simulink model "CAVE_MachE_sil_test_v2"  (R2019b)
settings: configuration reference "ConfigSetDesktopFixedStep" (kept outside this file)
PreLoadFcn:
  | VSS_BICYCLE=Simulink.Variant('Dual=0');
  | VSS_DUAL=Simulink.Variant('Dual=1');
  | Dual=1;
  | load('DriveCycle2.mat')
PostLoadFcn:
  | if any(exist('dsrtsu_mdlpostloadfcn', 'file') ~= 0), dsrtsu_mdlpostloadfcn('Execute', bdroot); end
InitFcn:
  | , if any(exist('dsmpb_private', 'file') ~= 0), dsmpb_private('dsmpb_mdlclblib', 'Init', bdroot); end,
  | load('DriveCycle2.mat')
model workspace (MAT data in the model file):
  Gas = 0.383333333333
values from neighbouring files (symbols this model uses):
  CoastDown =     [Run_Simulink.mat]
  limitedMCT =     [Run_Simulink.mat]
  MCT =     [Run_Simulink.mat]
  pMCT =     [Run_Simulink.mat]
  US06 =     [Run_Simulink.mat]
undefined symbols (not defined in the file or in its folder): AccelCmd, ActTqLF_Nm_, ActTqLR_Nm_, ActTqRF_Nm_, ActTqRR_Nm_, BattChargeLimitMaxPwr, BattChargeLimitSocBpts, BattChargeLimitTbl, BattChrgCapcty, BattDischargeLimitSocBpts, BattDischargeLimitTbl, BattDischargeMaxPwr, BattNumCellsParallel, BattNumCellsSeries, BattOpenVoltCapBpts, BattOpenVoltTbl, BattResistSocBpts, BattResistTbl, BattResistTempBpts, BrakeMaxPrs, BrakeMaxTrq, ChassisDistCg2FrontAxle, ChassisDistCg2RearAxle, ChassisVehMass, CltchCmd, DecelCmd, DiffRatio, DiscIntNeverNeededParam, EnvGravCnst, EnvPrs, EnvTemp, FuelSpecificGrav, GearCmd, h, InitStates, lgSw, MtrEffSpdBpts, MtrEffTbl, MtrEffTrqBpts, MtrPwrMax, MtrTrqMax, SteeringCmd, SupvsryCtrlRegenBrkCutOffTbl, SupvsryCtrlRegenSpdBpts, TestScnrioCycleNum, VEH
libraries: VSIGenLib x39, simulink x27, etargetslib x24, CarMaker4SL x8, vehdynlibtire x8, vehdynlibsuspension x7, vehdynlibtirecommon x7, autolibutils x5, autolibshared x5, VsrLibWheel x4, autolibpowerinfoutils x3, sharedtransform x3
(part 1 of 12)
PreSaveFcn:
  | , if any(exist('dsmpb_private', 'file') ~= 0), dsmpb_private('dsmpb_mdlclblib', 'PreSave', bdroot); end,
CloseFcn:
  | , if any(exist('dsmpb_private', 'file') ~= 0), dsmpb_private('dsmpb_mdlclblib', 'Close', bdroot); end,
settings Model: DataDictionary=DdPassengerEv.sldd  EnableAccessToBaseWorkspace=off  DSMPB_ID_DATA={'19138',struct('BlockId','c43ab22d-bd8f-46e8-9c1b-50244a2b4c3c','SignalIds',{{'677ec428-0e4b-4948-912c-2a0f547451ce'}}),'19214',struct('BlockId','c6d59404-7243-491d-a0f6-53a7c58573d2','SignalIds',{{'1bb5ce4d-6ca7-438d-a7c7-83dc6b8f8ba2','d23deae5-7b45-4d37-a8c2-65a1bc4ec57e','d73ea5da-e326-4b10-9ae8-bf6dd5d0d571','a3187cc6-40b5-42b9-9fee-06cfa4cf2657','616fd28a-17a3-40f5-a1a4-f6fdafbaa436'}})}  RTICANMMDATA=struct('GeneralSetupData',struct('modelroot','C:\GitDev\Anye\cave_carla_dev\Vehicles\VehicleProjects\Bolt_EV\System','generalsettings',struct('filesettings',struct('destfolder',struct('Name','RTICANMM_FILES','Check',1),'buildfolder',struct('Name','.','Check',1),'AbsDestfolder',struct('Name','C:\GitDev\Anye\cave_carla_dev\Vehicles\VehicleProjects\Bolt_EV\System\RTICANMM_FILES'),'AbsBuildfolder',struct('Name','C:\GitDev\Anye\cave_carla_dev\Vehicles\VehicleProjects\Bolt_EV\System'))),'options',struct('addpaths',1,'rmpaths',1,'addtrcexclusion',true,'cannavigator',struct('checkmonitoring',0),'show_usrtrc',0,'use_usrtrc',0),'advanced',struct('options',ones(1,100)),'MPSetup',{{}},'RTI',struct('Type','DSRT','Ver','4.2p1','Date','11-Feb-2020'),'modelname','CAVE_MachE_sil_test_v2','block','CAVE_MachE_sil_test_v2'))  DSRTSU_INTERNAL_RTIFPGA=150  PauseTimes=45  OrderedModelArguments=off  Creator=9bt  LastModifiedBy=RVDP
settings ConfigSetRef: SourceName=ConfigSetDesktopFixedStep

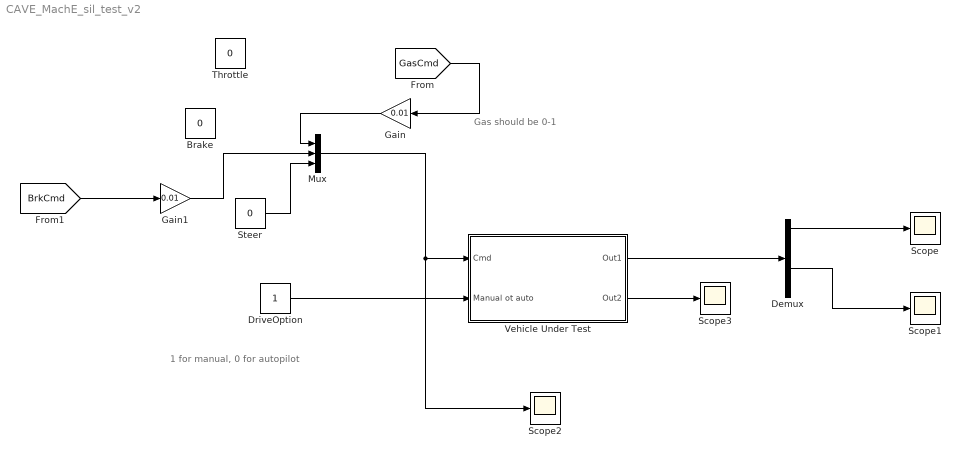
== system CAVE_MachE_sil_test_v2 ==
  note: 1 for manual, 0 for autopilot
  note: Gas should be 0-1
  Brake : Constant  Value=0
  Demux : Demux
  DriveOption : Constant
  Gain : Gain  Gain=0.01
  Gain1 : Gain  Gain=0.01
  Mux : Mux  Inputs=3
  Scope{,1..3} (4 alike) : Scope
  Steer : Constant  Value=0
  Throttle : Constant  Value=0
  Vehicle Under Test : Subsystem
  wires:
  Vehicle Under Test/1(Out1) -> Demux/1
  Demux/1 -> Scope/1
  Mux/1 -> Scope2/1, Vehicle Under Test/1(Cmd)
  Demux/3 -> Scope1/1
  Vehicle Under Test/2(Out2) -> Scope3/1
  DriveOption/1 -> Vehicle Under Test/2(Manual ot auto)
  [GasCmd] -> Gain/1
  [BrkCmd] -> Gain1/1
  Steer/1 -> Mux/3
  Gain1/1 -> Mux/2
  Gain/1 -> Mux/1

== system CAVE_MachE_sil_test_v2/Vehicle Under Test ==
  Cmd : Inport
  Manual ot auto : Inport  Port=2
  AccelCmdOutput_Anye : Terminator
  Ackerman steer : Lookup_n-D  NumberOfTableDimensions=1  BreakpointsForDimension1="[-0.446316297916244\t-0.442150786830951\t-0.437977161945005\t-0.433795286969319\t-0.429605025209166\t-0.425406239561593\t-0.421198792513030\t-0.416982546137136\t-0.412757362092861\t-0.408523101622746\t-0.404279625551461\t-0.400026794284603\t-0.395764467807732\t-0.391492505685692\t-0.387210767062193\t-0.382919110659678\t-0.378617394779480\t-0.374305477302279\t-0.369983215688866\t-0.365650466981227\t-0.361307087803951\t-0.356952934365975\t-0.352587862462675\t-0.348211727478321\t-0.343824384388886\t-0.339425687765245\t-0.335015491776758\t-0.330593650195247\t-0.326160016399396\t-0.321714443379563\t-0.317256783743034\t-0.312786889719717\t-0.308304613168298\t-0.303809805582871\t-0.299302318100048\t-0.294782001506567\t-0.290248706247410\t-0.285702282434450\t-0.281142579855627\t-0.276569447984685\t-0.271982735991464\t-0.267382292752788\t-0.262767966863931\t-0.258139606650706\t-0.253497060182174\t-0.248840175283994\t-0.244168799552432\t-0.239482780369037\t-0.234781964916014\t-0.230066200192295\t-0.225335333030331\t-0.220589210113630\t-0.215827677995039\t-0.211050583115807\t-0.206257771825433\t-0.201449090402323\t-0.196624385075265\t-0.191783502045761\t-0.186926287511198\t-0.182052587688919\t-0.177162248841170\t-0.172255117300976\t-0.167331039498945\t-0.162389861991014\t-0.157431431487183\t-0.152455594881217\t-0.147462199281363\t-0.142451092042095\t-0.137422120796894\t-0.132375133492088\t-0.127309978421782\t-0.122226504263869\t-0.117124560117169\t-0.112003995539695\t-0.106864660588066\t-0.101706405858090\t-0.0965290825265349\t-0.0913325423940914\t-0.0861166379295599\t-0.0808812223152671\t-0.0756261494937309\t-0.0703512742155897\t-0.0650564520888085\t-0.0597415396291770\t-0.0544063943121130\t-0.0490508746257825\t-0.0436748401255510\t-0.0382781514897739\t-0.0328606705769398\t-0.0274222604841732\t-0.0219627856071077\t-0.0164821117011354\t-0.0109801059440403\t-0.00545663700002112\t0\t0.00547767577609933\t0.0110656090794470\t0.0166755107772618\t0.0223075038233658\t0.0279617092740365\t0.0336382462142580\t0.0393372316825870\t0.0450587805946413\t0.0508030056652199\t0.0565700173290652\t0.0623599236602815\t0.0681728302904245\t0.0740088403252790\t0.0798680542603446\t0.0857505698950509\t0.0916564822457268\t0.0975858834573503\t0.103538862714108\t0.109515506148794\t0.115515896751090\t0.121540114274751\t0.127588235143750\t0.133660332357415\t0.139756475394610\t0.145876730117007\t0.152021158671496\t0.158189819391799\t0.164382766699339\t0.170600051003425\t0.176841718600822\t0.183107811574771\t0.189398367693541\t0.195713420308563\t0.202052998252265\t0.208417125735647\t0.214805822245717\t0.221219102442855\t0.227656976058216\t0.234119447791246\t0.240606517207442\t0.247118178636427\t0.253654421070478\t0.260215228063589\t0.266800577631217\t0.273410442150791\t0.280044788263140\t0.286703576774936\t0.293386762562311\t0.300094294475738\t0.306826115246357\t0.313582161393837\t0.320362363135953\t0.327166644299990\t0.333994922236136\t0.340847107733006\t0.347723104935443\t0.354622811264752\t0.361546117341510\t0.368492906911125\t0.375463056772267\t0.382456436708368\t0.389472909422305\t0.396512330474460\t0.403574548224288\t0.410659403775562\t0.417766730925451\t0.424896356117582\t0.432048098399246\t0.439221769382891\t0.446417173212069\t0.453634106531970\t0.460872358464695\t0.468131710589418\t0.475411936927561\t0.482712803933137\t0.490034070488372\t0.497375487904758\t0.504736799929627\t0.512117742758400\t0.519518045052588\t0.526937427963674\t0.534375605162959\t0.541832282877473\t0.549307159932028\t0.556799927797496\t0.564310270645373\t0.571837865408689\t0.579382381849329\t0.586943482631776\t0.594520823403350\t0.602114052880920\t0.609722812944144\t0.617346738735206\t0.624985458765058]"  Table="[-9.40000000000000\t-9.30000000000000\t-9.20000000000000\t-9.10000000000000\t-9\t-8.90000000000000\t-8.80000000000000\t-8.70000000000000\t-8.60000000000000\t-8.50000000000000\t-8.40000000000000\t-8.30000000000000\t-8.20000000000000\t-8.10000000000000\t-8\t-7.90000000000000\t-7.80000000000000\t-7.70000000000000\t-7.60000000000000\t-7.50000000000000\t-7.40000000000000\t-7.30000000000000\t-7.20000000000000\t-7.10000000000000\t-7\t-6.90000000000000\t-6.80000000000000\t-6.70000000000000\t-6.60000000000000\t-6.50000000000000\t-6.40000000000000\t-6.30000000000000\t-6.20000000000000\t-6.10000000000000\t-6\t-5.90000000000000\t-5.80000000000000\t-5.70000000000000\t-5.60000000000000\t-5.50000000000000\t-5.40000000000000\t-5.30000000000000\t-5.20000000000000\t-5.10000000000000\t-5\t-4.90000000000000\t-4.80000000000000\t-4.70000000000000\t-4.60000000000000\t-4.50000000000000\t-4.40000000000000\t-4.30000000000000\t-4.20000000000000\t-4.10000000000000\t-4\t-3.90000000000000\t-3.80000000000000\t-3.70000000000000\t-3.60000000000000\t-3.50000000000000\t-3.40000000000000\t-3.30000000000000\t-3.20000000000000\t-3.10000000000000\t-3\t-2.90000000000000\t-2.80000000000000\t-2.70000000000000\t-2.60000000000000\t-2.50000000000000\t-2.40000000000000\t-2.30000000000000\t-2.20000000000000\t-2.10000000000000\t-2\t-1.90000000000000\t-1.80000000000000\t-1.70000000000000\t-1.60000000000000\t-1.50000000000000\t-1.40000000000000\t-1.30000000000000\t-1.20000000000000\t-1.10000000000000\t-1\t-0.900000000000000\t-0.800000000000000\t-0.700000000000000\t-0.600000000000000\t-0.500000000000000\t-0.400000000000000\t-0.300000000000000\t-0.200000000000000\t-0.100000000000000\t0\t0.100000000000000\t0.200000000000000\t0.300000000000000\t0.400000000000000\t0.500000000000000\t0.600000000000000\t0.700000000000000\t0.800000000000000\t0.900000000000000\t1\t1.10000000000000\t1.20000000000000\t1.30000000000000\t1.40000000000000\t1.50000000000000\t1.60000000000000\t1.70000000000000\t1.80000000000000\t1.90000000000000\t2\t2.10000000000000\t2.20000000000000\t2.30000000000000\t2.40000000000000\t2.50000000000000\t2.60000000000000\t2.70000000000000\t2.80000000000000\t2.90000000000000\t3\t3.10000000000000\t3.20000000000000\t3.30000000000000\t3.40000000000000\t3.50000000000000\t3.60000000000000\t3.70000000000000\t3.80000000000000\t3.90000000000000\t4\t4.10000000000000\t4.20000000000000\t4.30000000000000\t4.40000000000000\t4.50000000000000\t4.60000000000000\t4.70000000000000\t4.80000000000000\t4.90000000000000\t5\t5.10000000000000\t5.20000000000000\t5.30000000000000\t5.40000000000000\t5.50000000000000\t5.60000000000000\t5.70000000000000\t5.80000000000000\t5.90000000000000\t6\t6.10000000000000\t6.20000000000000\t6.30000000000000\t6.40000000000000\t6.50000000000000\t6.60000000000000\t6.70000000000000\t6.80000000000000\t6.90000000000000\t7\t7.10000000000000\t7.20000000000000\t7.30000000000000\t7.40000000000000\t7.50000000000000\t7.60000000000000\t7.70000000000000\t7.80000000000000\t7.90000000000000\t8\t8.10000000000000\t8.20000000000000\t8.30000000000000\t8.40000000000000\t8.50000000000000\t8.60000000000000\t8.70000000000000\t8.80000000000000\t8.90000000000000\t9\t9.10000000000000\t9.20000000000000\t9.30000000000000\t9.40000000000000]"  InternalRulePriority=Speed  RndMeth=Simplest  InputSameDT=on
  Bus Creator : BusCreator  Inputs=AccelCmd,DecelCmd,GearCmd,CltchCmd,lgSw,SteeringCmd
  Bus Creator1 : BusCreator  Inputs=8
  Bus Creator2 : BusCreator  Inputs=2
  Bus Selector : BusSelector  OutputSignals=Veh.Chassis.X,Veh.Chassis.Y,Veh.Chassis.psi,Veh.Batt.BattSoc,Veh.Batt.BattCurr,Veh.Batt.BattVolt,Veh.Diff.Axl1.Axl1Trq,Veh.Chassis.VehSpd
  Clock : Clock
  Constant : Constant  Value=0
  Constant1 : Constant  Value=0  SampleTime=0.001
  Constant2 : Constant
  Constant3 : Constant  Value=0
  Constant4 : Constant
  Constant6 : Constant  Value=0.5  SampleTime=0.001
  Demux : Demux  Outputs=3
  EV Bolt Steer : Lookup_n-D  NumberOfTableDimensions=1  BreakpointsForDimension1="[-0.541571931581492\t-0.535619550629112\t-0.529667169676731\t-0.523714788724350\t-0.517762407771969\t-0.511810026819588\t-0.505857645867207\t-0.499905264914826\t-0.493952883962445\t-0.488000503010064\t-0.482048122057683\t-0.476095741105302\t-0.470143360152921\t-0.464190979200541\t-0.458238598248160\t-0.452286217295779\t-0.446333836343398\t-0.440381455391017\t-0.434429074438636\t-0.428476693486255\t-0.422524312533874\t-0.416571931581493\t-0.410619550629112\t-0.404667169676731\t-0.398714788724350\t-0.392762407771969\t-0.386810026819588\t-0.380857645867207\t-0.374905264914826\t-0.368952883962445\t-0.363000503010064\t-0.357048122057683\t-0.351095741105302\t-0.345143360152921\t-0.339190979200541\t-0.333238598248160\t-0.327286217295779\t-0.321333836343398\t-0.315381455391017\t-0.309429074438636\t-0.303476693486255\t-0.297524312533874\t-0.291571931581493\t-0.285619550629112\t-0.279667169676731\t-0.273714788724350\t-0.267762407771969\t-0.261810026819588\t-0.255857645867207\t-0.249905264914826\t-0.243952883962445\t-0.238000503010065\t-0.232048122057684\t-0.226095741105303\t-0.220143360152922\t-0.214190979200541\t-0.208238598248160\t-0.202286217295779\t-0.196333836343398\t-0.190381455391017\t-0.184429074438636\t-0.178476693486255\t-0.172524312533874\t-0.166571931581493\t-0.160619550629112\t-0.154667169676731\t-0.148714788724350\t-0.142762407771969\t-0.136810026819588\t-0.130857645867207\t-0.124905264914826\t-0.118952883962445\t-0.113000503010064\t-0.107048122057683\t-0.101095741105303\t-0.0951433601529216\t-0.0891909792005406\t-0.0832385982481596\t-0.0772862172957787\t-0.0713338363433977\t-0.0653814553910168\t-0.0594290744386358\t-0.0534766934862548\t-0.0475243125338739\t-0.0415719315814929\t-0.0356195506291120\t-0.0296671696767310\t-0.0237147887243500\t-0.0177624077719691\t-0.0118100268195881\t-0.00585764586720720\t0\t0.00585764586720720\t0.0118100268195881\t0.0177624077719691\t0.0237147887243500\t0.0296671696767310\t0.0356195506291120\t0.0415719315814929\t0.0475243125338739\t0.0534766934862548\t0.0594290744386358\t0.0653814553910168\t0.0713338363433977\t0.0772862172957787\t0.0832385982481596\t0.0891909792005406\t0.0951433601529216\t0.101095741105303\t0.107048122057683\t0.113000503010064\t0.118952883962445\t0.124905264914826\t0.130857645867207\t0.136810026819588\t0.142762407771969\t0.148714788724350\t0.154667169676731\t0.160619550629112\t0.166571931581493\t0.172524312533874\t0.178476693486255\t0.184429074438636\t0.190381455391017\t0.196333836343398\t0.202286217295779\t0.208238598248160\t0.214190979200541\t0.220143360152922\t0.226095741105303\t0.232048122057684\t0.238000503010065\t0.243952883962445\t0.249905264914826\t0.255857645867207\t0.261810026819588\t0.267762407771969\t0.273714788724350\t0.279667169676731\t0.285619550629112\t0.291571931581493\t0.297524312533874\t0.303476693486255\t0.309429074438636\t0.315381455391017\t0.321333836343398\t0.327286217295779\t0.333238598248160\t0.339190979200541\t0.345143360152921\t0.351095741105302\t0.357048122057683\t0.363000503010064\t0.368952883962445\t0.374905264914826\t0.380857645867207\t0.386810026819588\t0.392762407771969\t0.398714788724350\t0.404667169676731\t0.410619550629112\t0.416571931581493\t0.422524312533874\t0.428476693486255\t0.434429074438636\t0.440381455391017\t0.446333836343398\t0.452286217295779\t0.458238598248160\t0.464190979200541\t0.470143360152921\t0.476095741105302\t0.482048122057683\t0.488000503010064\t0.493952883962445\t0.499905264914826\t0.505857645867207\t0.511810026819588\t0.517762407771969\t0.523714788724350\t0.529667169676731\t0.535619550629112\t0.541571931581492]"  Table="[-9.10000000000000\t-9\t-8.90000000000000\t-8.80000000000000\t-8.70000000000000\t-8.60000000000000\t-8.50000000000000\t-8.40000000000000\t-8.30000000000000\t-8.20000000000000\t-8.10000000000000\t-8\t-7.90000000000000\t-7.80000000000000\t-7.70000000000000\t-7.60000000000000\t-7.50000000000000\t-7.40000000000000\t-7.30000000000000\t-7.20000000000000\t-7.10000000000000\t-7\t-6.90000000000000\t-6.80000000000000\t-6.70000000000000\t-6.60000000000000\t-6.50000000000000\t-6.40000000000000\t-6.30000000000000\t-6.20000000000000\t-6.10000000000000\t-6\t-5.90000000000000\t-5.80000000000000\t-5.70000000000000\t-5.60000000000000\t-5.50000000000000\t-5.40000000000000\t-5.30000000000000\t-5.20000000000000\t-5.10000000000000\t-5\t-4.90000000000000\t-4.80000000000000\t-4.70000000000000\t-4.60000000000000\t-4.50000000000000\t-4.40000000000000\t-4.30000000000000\t-4.20000000000000\t-4.10000000000000\t-4\t-3.90000000000000\t-3.80000000000000\t-3.70000000000000\t-3.60000000000000\t-3.50000000000000\t-3.40000000000000\t-3.30000000000000\t-3.20000000000000\t-3.10000000000000\t-3\t-2.90000000000000\t-2.80000000000000\t-2.70000000000000\t-2.60000000000000\t-2.50000000000000\t-2.40000000000000\t-2.30000000000000\t-2.20000000000000\t-2.10000000000000\t-2\t-1.90000000000000\t-1.80000000000000\t-1.70000000000000\t-1.60000000000000\t-1.50000000000000\t-1.40000000000000\t-1.30000000000000\t-1.20000000000000\t-1.10000000000000\t-1\t-0.900000000000000\t-0.800000000000000\t-0.700000000000000\t-0.600000000000000\t-0.500000000000000\t-0.400000000000000\t-0.300000000000000\t-0.200000000000000\t-0.100000000000000\t0\t0.100000000000000\t0.200000000000000\t0.300000000000000\t0.400000000000000\t0.500000000000000\t0.600000000000000\t0.700000000000000\t0.800000000000000\t0.900000000000000\t1\t1.10000000000000\t1.20000000000000\t1.30000000000000\t1.40000000000000\t1.50000000000000\t1.60000000000000\t1.70000000000000\t1.80000000000000\t1.90000000000000\t2\t2.10000000000000\t2.20000000000000\t2.30000000000000\t2.40000000000000\t2.50000000000000\t2.60000000000000\t2.70000000000000\t2.80000000000000\t2.90000000000000\t3\t3.10000000000000\t3.20000000000000\t3.30000000000000\t3.40000000000000\t3.50000000000000\t3.60000000000000\t3.70000000000000\t3.80000000000000\t3.90000000000000\t4\t4.10000000000000\t4.20000000000000\t4.30000000000000\t4.40000000000000\t4.50000000000000\t4.60000000000000\t4.70000000000000\t4.80000000000000\t4.90000000000000\t5\t5.10000000000000\t5.20000000000000\t5.30000000000000\t5.40000000000000\t5.50000000000000\t5.60000000000000\t5.70000000000000\t5.80000000000000\t5.90000000000000\t6\t6.10000000000000\t6.20000000000000\t6.30000000000000\t6.40000000000000\t6.50000000000000\t6.60000000000000\t6.70000000000000\t6.80000000000000\t6.90000000000000\t7\t7.10000000000000\t7.20000000000000\t7.30000000000000\t7.40000000000000\t7.50000000000000\t7.60000000000000\t7.70000000000000\t7.80000000000000\t7.90000000000000\t8\t8.10000000000000\t8.20000000000000\t8.30000000000000\t8.40000000000000\t8.50000000000000\t8.60000000000000\t8.70000000000000\t8.80000000000000\t8.90000000000000\t9\t9.10000000000000]"  InternalRulePriority=Speed  RndMeth=Simplest  InputSameDT=on
  Environment : Subsystem
  Monitor : Subsystem
  Step : Step  Time=3  After=0
  Switch : Switch  Criteria=u2 > Threshold
  Switch1 : Switch  Criteria=u2 > Threshold
  Switch2 : Switch  Criteria=u2 > Threshold
  To Workspace : ToWorkspace  VariableName=EvBoltCalib  SaveFormat=Structure With Time  SampleTime=-1
  Vector Concatenate : Concatenate  NumInputs=4
  Vehicle : Subsystem
  Out1 : Outport
  Out2 : Outport  Port=2
  wires:
  Bus Creator2/1 -> Bus Selector/1, Monitor/1(Monitor)  "SimMonitor"
  Vehicle/1(Veh) -> [Veh]
  [Driver] -> Bus Creator2/1  "Driver"
  Constant3/1 -> Bus Creator/4  "CltchCmd"
  Cmd/1 -> Demux/1
  Bus Creator/1 -> [Driver], Vehicle/2(Driver)
  [Veh] -> Bus Creator2/2  "Veh"
  Environment/1(Env) -> Vehicle/1(Env)
  Constant/1 -> Environment/1(Grade)
  Constant4/1 -> Bus Creator/5  "lgSw"
  Bus Creator1/1 -> To Workspace/1
  Constant2/1 -> Bus Creator/3  "GearCmd"
  Vector Concatenate/1 -> Out1/1
  Clock/1 -> Vector Concatenate/4, Bus Creator1/8
  Bus Selector/1 -> Vector Concatenate/1, Bus Creator1/1  "<X>"
  Bus Selector/2 -> Vector Concatenate/2, Bus Creator1/2  "<Y>"
  Bus Selector/3 -> Vector Concatenate/3, Bus Creator1/3  "<psi>"
  Bus Selector/4 -> Bus Creator1/4  "<BattSoc>"
  Bus Selector/5 -> Bus Creator1/5  "<BattCurr>"
  Bus Selector/6 -> Bus Creator1/6  "<BattVolt>"
  Bus Selector/7 -> Bus Creator1/7  "<Axl1Trq>"
  Bus Selector/8 -> Out2/1  "<VehSpd>"
  EV Bolt Steer/1 -> Bus Creator/6  "SteeringCmd"
  Switch2/1 -> EV Bolt Steer/1
  Switch/1 -> Bus Creator/1, AccelCmdOutput_Anye/1  "AccelCmd"
  Switch1/1 -> Bus Creator/2  "DecelCmd"
  Manual ot auto/1 -> [Autopilot]
  [Autopilot] -> Switch2/2, Switch1/2, Switch/2
  Step/1 -> Switch/3  "AccelCmd"
  Demux/1 -> Switch/1  "AccelCmd"
  Constant6/1 -> Switch1/3  "DecelCmd"
  Demux/2 -> Switch1/1  "DecelCmd"
  Constant1/1 -> Switch2/3
  Demux/3 -> Switch2/1

== system CAVE_MachE_sil_test_v2/Vehicle Under Test/Environment ==
  Grade : Inport
  Friction : Constant  Value=ones(4,1).*1
  Ground Feedback : Subsystem  VariantControlMode=Label  Variant=on  LabelModeActiveChoice=0
  Ground Z Level : Constant  Value=zeros(4,1)
  Subsystem : Subsystem
  Subsystem1 : Subsystem
      mask Display: disp('')
  Env : Outport
  wires:
  Subsystem/3(WindVel) -> Subsystem1/3(WindVel)
  Subsystem/2(EnvTemp) -> Subsystem1/2(EnvTemp)
  Subsystem/4(RoadGrade) -> Subsystem1/4(RoadGrade)
  Subsystem/1(EnvPrs) -> Subsystem1/1(EnvPrs)
  Subsystem1/1(Env) -> Env/1
  Friction/1 -> Ground Feedback/1(Friction)
  Ground Feedback/1(Ground) -> Subsystem1/5(GroundBus)  "Gnd"
  Ground Z Level/1 -> Ground Feedback/2(Ground Z Level)
  Grade/1 -> Subsystem/1(Grade)

== system CAVE_MachE_sil_test_v2/Vehicle Under Test/Monitor ==
  Monitor : Inport
  Calculate Fuel MPG : Subsystem  Commented=on
  Calculate Powertrain Energy : Subsystem
  Terminator : Terminator
  Terminator3 : Terminator
  wires:
  Calculate Fuel MPG/1(FuelEconMPG) -> Terminator/1  "FuelEconMpg"
  Monitor/1 -> Calculate Powertrain Energy/1(Monitor), Calculate Fuel MPG/1(Monitor)
  Calculate Powertrain Energy/1(TransEnrgyOutkWh) -> Terminator3/1  "DiffEnrgyInkWh"

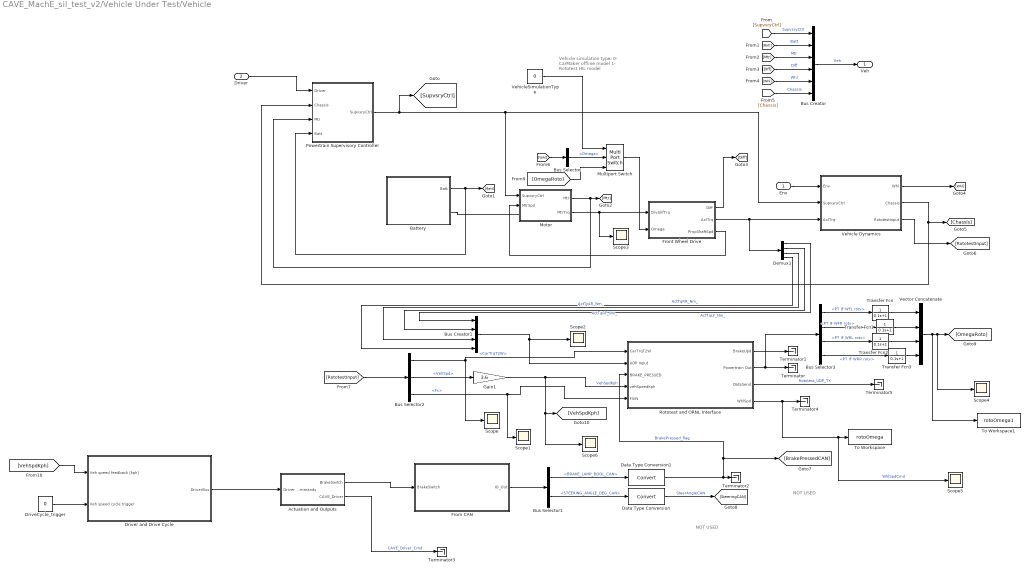
== system CAVE_MachE_sil_test_v2/Vehicle Under Test/Vehicle ==
  note: Vehicle simulation type:
      | 0- CarMaker offline model
      | 1- Rototest HIL model
  note: NOT USED
  note: NOT USED
  Env : Inport
  Driver : Inport  Port=2
  Actuation and Outputs : Subsystem
  Battery : Subsystem
  Bus Creator : BusCreator  Inputs=6
  Bus Creator1 : BusCreator  Inputs=ActTqLF_Nm_,ActTqRF_Nm_,ActTqLR_Nm_,ActTqRR_Nm_
  Bus Selector : BusSelector  OutputSignals=Omega
  Bus Selector1 : BusSelector  OutputSignals=BRAKE_LAMP_BOOL_CAN,STEERING_ANGLE_DEG_CAN
  Bus Selector2 : BusSelector  OutputSignals=CarTrqT2W,VehSpd,Fx
  Bus Selector3 : BusSelector  OutputSignals=PT IF WFL rotv,PT IF WFR rotv,PT IF WRL rotv,PT IF WRR rotv
  Data Type Conversion : DataTypeConversion
  Data Type Conversion1 : DataTypeConversion
  Demux1 : Demux
  DriveCycle_trigger : Constant  Value=0
  Driver and Drive Cycle : Subsystem  TreatAsAtomicUnit=on
  From CAN : Subsystem
  Front Wheel Drive : Subsystem  VariantControlMode=Label  Variant=on  VariantControl=1  LabelModeActiveChoice=Choice
  Gain1 : Gain  Gain=3.6
  Motor : Subsystem
  Multiport Switch : MultiPortSwitch  DataPortOrder=Zero-based contiguous  Inputs=2  zeroidx=on
  "Powertrain Supervisory Controller " : Subsystem  AncestorBlock=LibPtSupervisoryCtrl/Powertrain Supervisory Controller
  Rototest and ORNL Interface : Subsystem
  Scope{,1..6} (7 alike) : Scope
  Terminator{,1..5} (6 alike) : Terminator
  To Workspace : ToWorkspace  VariableName=rotoOmega  SampleTime=-1
      settings: Save2DSignal=2-D array (concatenate along first dimension)
  To Workspace1 : ToWorkspace  VariableName=rotoOmega1  SampleTime=-1
      settings: Save2DSignal=2-D array (concatenate along first dimension)
  Transfer Fcn{,1..3} (4 alike) : TransferFcn  Denominator=[0.1 1]
  Vector Concatenate : Concatenate  NumInputs=4
  Vehicle Dynamics : Subsystem  VariantControlMode=Label  Variant=on  LabelModeActiveChoice=Veh14DOF  mask{VehDynSel=Vehicle 14DOF}
      mask prompts: VehDynSel "Select the driver"
      mask init:
      | choice = get_param(gcb,'VehDynSel');
      | curBlk = gcb;
      | oldVariant = get_param(gcb,'LabelModeActiveChoice');
      | switch choice
      |     case 'Vehicle Longitudinal'
      |         set_param(curBlk, 'LabelModeActiveChoice', 'VehLong');
      | %     case 'Vehicle 3DOF'   
      | %         set_param(curBlk, 'LabelModeActiveChoice', 'Veh3DOF');
      |     case 'Vehicle 7DOF'   
      |         set_param(curBlk, 'LabelModeActiveChoice', 'Veh7DOF');
      |     case 'Vehicle 14DOF'   
      |         set_param(curBlk, 'LabelModeActiveChoice', 'Veh14DOF');
      | end
      mask TypeOptions VehDynSel: Vehicle Longitudinal | Vehicle 7DOF | Vehicle 14DOF
  VehicleSimulationType : Constant  Value=0
  Veh : Outport
  wires:
  "Powertrain Supervisory Controller "/1(SupvsryCtrl) -> Vehicle Dynamics/2(SupvsryCtrl), Motor/1(SupvsryCtrl), [SupvsryCtrl]
  Driver/1 -> "Powertrain Supervisory Controller "/1(Driver)
  Bus Creator/1 -> Veh/1  "Veh"
  [SupvsryCtrl] -> Bus Creator/1  "SupvsryCtrl"
  [Batt] -> Bus Creator/2  "Batt"
  [Mtr] -> Bus Creator/3  "Mtr"
  [Whl] -> Bus Creator/5  "Whl"
  [Chassis] -> Bus Creator/6  "Chassis"
  Battery/1(Batt) -> "Powertrain Supervisory Controller "/4(Batt), [Batt]
  Motor/1(Mtr) -> "Powertrain Supervisory Controller "/3(Mtr), [Mtr]
  Env/1 -> Vehicle Dynamics/1(Env)
  Vehicle Dynamics/2(Chassis) -> "Powertrain Supervisory Controller "/2(Chassis), [Chassis]
  Vehicle Dynamics/1(Whl) -> [Whl]
  [Whl] -> Bus Selector/1
  [Diff] -> Bus Creator/4  "Diff"
  Front Wheel Drive/1(Diff) -> [Diff]
  Front Wheel Drive/3(PropShaftSpd) -> Motor/2(MtrSpd)
  Motor/2(MtrTrq) -> Scope3/1, Front Wheel Drive/1(DrvShfTrq)
  Front Wheel Drive/2(AxlTrq) -> Demux1/1, Vehicle Dynamics/3(AxlTrq)
  Vehicle Dynamics/3(RototestInput) -> [RototestInput]
  VehicleSimulationType/1 -> Multiport Switch/1
  Bus Selector/1 -> Multiport Switch/2  "<Omega>"
  [OmegaRoto] -> Multiport Switch/3
  Multiport Switch/1 -> Front Wheel Drive/2(Omega)
  Bus Selector3/2 -> Transfer Fcn1/1  "<PT IF WFR rotv>"
  Rototest and ORNL Interface/2(Powertrain Out) -> Bus Selector3/1, Terminator/1
  Bus Selector3/3 -> Transfer Fcn2/1  "<PT IF WRL rotv>"
  Bus Selector3/1 -> Transfer Fcn/1  "<PT IF WFL rotv>"
  Rototest and ORNL Interface/3(DataSend) -> Terminator5/1  "Rototest_UDP_TX"
  Gain1/1 -> Scope6/1, [VehSpdKph], Rototest and ORNL Interface/4(vehSpeedKph)  "VehSpdKph"
  Bus Selector3/4 -> Transfer Fcn3/1  "<PT IF WRR rotv>"
  Bus Creator1/1 -> Scope2/1, Rototest and ORNL Interface/2(UDP Input)
  Rototest and ORNL Interface/4(WhlSpd) -> Scope5/1, To Workspace/1, Terminator4/1  "WhlSpdCmd"
  Rototest and ORNL Interface/1(BrakeUpd) -> Terminator1/1
  Bus Selector2/3 -> Rototest and ORNL Interface/5(FXIN), Scope1/1  "<Fx>"
  [RototestInput] -> Bus Selector2/1
  Bus Selector2/2 -> Gain1/1  "<VehSpd>"
  Bus Selector2/1 -> Rototest and ORNL Interface/1(CarTrqT2W), Scope/1  "<CarTrqT2W>"
  Demux1/3 -> Bus Creator1/3  "ActTqLR_Nm_"
  Demux1/4 -> Bus Creator1/4  "ActTqRR_Nm_"
  Demux1/2 -> Bus Creator1/2  "ActTqRF_Nm_"
  Demux1/1 -> Bus Creator1/1  "ActTqLF_Nm_"
  Vector Concatenate/1 -> To Workspace1/1, Scope4/1, [OmegaRoto]
  Transfer Fcn/1 -> Vector Concatenate/1
  Transfer Fcn1/1 -> Vector Concatenate/2
  Transfer Fcn2/1 -> Vector Concatenate/3
  Transfer Fcn3/1 -> Vector Concatenate/4
  Data Type Conversion1/1 -> Rototest and ORNL Interface/3(BRAKE_PRESSED), [BrakePressedCAN], Terminator2/1  "BrakePressed_flag"
  [VehSpdKph] -> Driver and Drive Cycle/1(Veh speed feedback [kph])
  DriveCycle_trigger/1 -> Driver and Drive Cycle/2(Veh speed cycle trigger)
  From CAN/1(IO_Out) -> Bus Selector1/1
  Bus Selector1/2 -> Data Type Conversion/1  "<STEERING_ANGLE_DEG_CAN>"
  Data Type Conversion/1 -> [SteeringCAN]  "SteerAngleCAN"
  Actuation and Outputs/1(BrakeSwitch) -> From CAN/1(BrakeSwitch)
  Driver and Drive Cycle/1(DriverBus) -> Actuation and Outputs/1(Driver Commands)
  Actuation and Outputs/2(CAVE_Driver) -> Terminator3/1  "CAVE_Driver_Cmd"
  Bus Selector1/1 -> Data Type Conversion1/1  "<BRAKE_LAMP_BOOL_CAN>"
  connections:
  Battery/RConn1 -- Motor/LConn1

== system CAVE_MachE_sil_test_v2/Vehicle Under Test/Environment/Ground Feedback ==
  note: 1) Add Subsystem or Model blocks as valid variant choices.
      | 2) You cannot connect blocks at this level. At simulation, connectivity is automatically
      | determined, based on the active variant and port name matching.
  Friction : Inport
  Ground Z Level : Inport  Port=2
  3D Engine : Subsystem  VariantControl=1
  Constant : Subsystem  VariantControl=0
  Ground : Outport  VectorParamsAs1DForOutWhenUnconnected=off

== system CAVE_MachE_sil_test_v2/Vehicle Under Test/Environment/Subsystem ==
  Grade : Inport
  Constant : Constant  Value=EnvPrs
  Constant1 : Constant  Value=EnvTemp
  Constant2 : Constant  Value=0
  Constant3 : Constant  Value=0
  Constant4 : Constant  Value=0
  Signal Specification : SignalSpecification  Unit=Pa
  Signal Specification1 : SignalSpecification  Unit=K
  Signal Specification2 : SignalSpecification  Unit=rad
  Signal Specification3 : SignalSpecification  Unit=m/s
  Signal Specification4 : SignalSpecification  Unit=m/s
  Signal Specification5 : SignalSpecification  Unit=m/s
  Vector Concatenate : Concatenate  NumInputs=3
  EnvPrs : Outport
  EnvTemp : Outport  Port=2
  WindVel : Outport  Port=3
  RoadGrade : Outport  Port=4
  wires:
  Constant/1 -> Signal Specification/1
  Constant2/1 -> Signal Specification3/1
  Constant1/1 -> Signal Specification1/1
  Grade/1 -> Signal Specification2/1
  Signal Specification/1 -> EnvPrs/1
  Signal Specification1/1 -> EnvTemp/1
  Signal Specification2/1 -> RoadGrade/1
  Vector Concatenate/1 -> WindVel/1
  Signal Specification3/1 -> Vector Concatenate/1  "WindX"
  Constant3/1 -> Signal Specification4/1
  Constant4/1 -> Signal Specification5/1
  Signal Specification4/1 -> Vector Concatenate/2  "WindY"
  Signal Specification5/1 -> Vector Concatenate/3  "WindZ"

== system CAVE_MachE_sil_test_v2/Vehicle Under Test/Environment/Subsystem1 ==
  EnvPrs : Inport
  EnvTemp : Inport  Port=2
  WindVel : Inport  Port=3
  RoadGrade : Inport  Port=4
  GroundBus : Inport  Port=5
  Bus Creator : BusCreator  Inputs=5
  Env : Outport
  wires:
  EnvPrs/1 -> Bus Creator/1  "EnvPrs"
  EnvTemp/1 -> Bus Creator/2  "EnvTemp"
  Bus Creator/1 -> Env/1  "Env"
  WindVel/1 -> Bus Creator/3  "WindVel"
  RoadGrade/1 -> Bus Creator/4  "RoadGrade"
  GroundBus/1 -> Bus Creator/5  "GndBus"

== system CAVE_MachE_sil_test_v2/Vehicle Under Test/Monitor/Calculate Fuel MPG ==
  Monitor : Inport
  Bus Selector : BusSelector  OutputSignals=Veh.Chassis.VehDist,Veh.Batt.EngPlant.FuellMassFlw
  Constant : Constant  Value=FuelSpecificGrav
  Density of Water : Gain  Gain=997
  Divide : Product  Inputs=*/
  Divide1 : Product  Inputs=*/
  Integrator : Integrator
  Saturation : Saturate  UpperLimit=inf  LowerLimit=1e-7
  Signal Specification : SignalSpecification  Unit=mi
  Signal Specification1 : SignalSpecification  Unit=m^3
  Signal Specification2 : SignalSpecification  Unit=gal
  Unit Conversion : UnitConversion
  Unit Conversion1 : UnitConversion
  FuelEconMPG : Outport
  wires:
  Divide1/1 -> FuelEconMPG/1  "FuelEconMPG"
  Divide/1 -> Signal Specification1/1
  Unit Conversion1/1 -> Signal Specification2/1
  Signal Specification2/1 -> Saturation/1
  Unit Conversion/1 -> Signal Specification/1
  Bus Selector/1 -> Unit Conversion/1  "<VehDist>"
  Bus Selector/2 -> Integrator/1  "<FuellMassFlw>"
  Integrator/1 -> Divide/1  "FuelMass"
  Density of Water/1 -> Divide/2
  Saturation/1 -> Divide1/2  "FuelVolume"
  Constant/1 -> Density of Water/1
  Signal Specification1/1 -> Unit Conversion1/1
  Monitor/1 -> Bus Selector/1
  Signal Specification/1 -> Divide1/1  "VehDistMiles"

== system CAVE_MachE_sil_test_v2/Vehicle Under Test/Monitor/Calculate Powertrain Energy ==
  Monitor : Inport
  Bus Selector2 : BusSelector  OutputSignals=Veh.Diff.PwrInfo.PwrTrnsfrd.PwrTrnsfrd.PwrDriveshft
  Integrator : Integrator
  Signal Specification : SignalSpecification  Unit=J
  Signal Specification1 : SignalSpecification  Unit=kW*h
  Unit Conversion : UnitConversion
  TransEnrgyOutkWh : Outport
  wires:
  Unit Conversion/1 -> Signal Specification1/1
  Integrator/1 -> Signal Specification/1  "EnrgyTrans"
  Signal Specification/1 -> Unit Conversion/1
  Signal Specification1/1 -> TransEnrgyOutkWh/1
  Monitor/1 -> Bus Selector2/1
  Bus Selector2/1 -> Integrator/1  "<PwrDriveshft>"

== system CAVE_MachE_sil_test_v2/Vehicle Under Test/Vehicle/Actuation and Outputs ==
  note: Driver Commands are [0,100] for both pedal and brake
  Driver Commands : Inport
  APP : Constant  Value=0
  AR_limit : Saturate  UpperLimit=100  LowerLimit=0
  BR_command_0to100 : Constant  Value=0
  BR_limit : Saturate  UpperLimit=100  LowerLimit=0
  Bus Creator : BusCreator  Inputs=2
  Bus Selector1 : BusSelector  OutputSignals=AccelPedalCmd
  Bus Selector3 : BusSelector  OutputSignals=BrakePedalCmd
  Constant{,1..3} (4 alike) : Constant  Value=0
  Min threshold for Brake switch : Constant  Value=0
  Multiport Switch1 : MultiPortSwitch  Inputs=4
  Multiport Switch2 : MultiPortSwitch  Inputs=4
  Pedal Robot Control Selection : Constant  Value=2
  Relational Operator : RelationalOperator  Operator=>  OutDataTypeStr=boolean  RndMeth=Nearest
  Terminator : Terminator
  Terminator1 : Terminator
  bped2br_N : Lookup_n-D  NumberOfTableDimensions=1  BreakpointsForDimension1=[0 0.1 0.2 100]  Table=[0 0 25 100]  InternalRulePriority=Speed  RndMeth=Simplest  InputSameDT=on
  BrakeSwitch : Outport  VectorParamsAs1DForOutWhenUnconnected=off
  CAVE_Driver : Outport  Port=2
  tag scope: BrkCmd=global, GasCmd=global
  wires:
  Multiport Switch1/1 -> AR_limit/1
  APP/1 -> Multiport Switch1/2
  Bus Selector1/1 -> Multiport Switch1/3  "<AccelPedalCmd>"
  Multiport Switch2/1 -> BR_limit/1
  Driver Commands/1 -> Bus Selector3/1, Bus Selector1/1
  Pedal Robot Control Selection/1 -> Multiport Switch1/1, Multiport Switch2/1
  BR_command_0to100/1 -> Multiport Switch2/2
  Bus Selector3/1 -> Multiport Switch2/3  "<BrakePedalCmd>"
  bped2br_N/1 -> Terminator1/1
  Min threshold for Brake switch/1 -> Relational Operator/2
  Relational Operator/1 -> BrakeSwitch/1  "BrakeSwitch"
  Constant/1 -> Multiport Switch1/5
  Constant1/1 -> Multiport Switch2/5
  Bus Creator/1 -> CAVE_Driver/1
  AR_limit/1 -> Terminator/1, Bus Creator/1, [GasCmd]  "AccelPedalCmd_pct"
  BR_limit/1 -> [BrkCmd], Bus Creator/2, Relational Operator/1, bped2br_N/1  "BrakePedalCmd_pct"
  Constant2/1 -> Multiport Switch1/4
  Constant3/1 -> Multiport Switch2/4

== system CAVE_MachE_sil_test_v2/Vehicle Under Test/Vehicle/Battery ==
  Battery : Subsystem
  Subsystem1 : Subsystem
      mask Display: disp('')
  BattOut : PMIOPort  Side=Right
  Batt : Outport
  wires:
  Battery/1(BattSoc) -> Subsystem1/1(BattSoc)
  Battery/2(BattCurr) -> Subsystem1/2(BattCurr)
  Battery/3(BattVolt) -> Subsystem1/3(BattVolt)
  Subsystem1/1(Batt) -> Batt/1
  connections:
  BattOut/RConn1 -- Battery/RConn1

== system CAVE_MachE_sil_test_v2/Vehicle Under Test/Vehicle/Driver and Drive Cycle ==
  Veh speed feedback [kph] : Inport
  Veh speed cycle trigger : Inport  Port=2
  Add : Sum
  CoastDown : Lookup_n-D  NumberOfTableDimensions=1  BreakpointsForDimension1=CoastDown.Time  Table=CoastDown.Speed  InternalRulePriority=Speed  RndMeth=Simplest  InputSameDT=on
  Constant : Constant  Value=0
  Data Type Conversion11 : DataTypeConversion  OutDataTypeStr=double  LockScale=on
  DriveCycleSelect : Constant
  Driver and PI with FF Control : Subsystem
  Gain : Gain  Gain=1/1.609
  Gain1 : Gain  Gain=1/1.609
  Get Cycle Clock Time : Subsystem
  MCT : Lookup_n-D  NumberOfTableDimensions=1  BreakpointsForDimension1=MCT.Time  Table=MCT.Speed  InternalRulePriority=Speed  RndMeth=Simplest  InputSameDT=on
  ManSpd : Constant  Value=0
  ManSpdSel : Constant
  Multiport Switch : MultiPortSwitch  Inputs=5
  Multiport Switch1 : MultiPortSwitch  Inputs=4
  Pulse Generator : DiscretePulseGenerator  PulseType=Time based  Amplitude=5  Period=25  PulseWidth=40  PhaseDelay=2
  Rate Limiter : RateLimiter  RisingSlewLimit=3  FallingSlewLimit=-3  SampleTimeMode=inherited
  Scope : Scope  NumInputPorts=2
  Terminator : Terminator
  Terminator1 : Terminator
  US06 : Lookup_n-D  NumberOfTableDimensions=1  BreakpointsForDimension1=US06.Time  Table=US06.Speed  InternalRulePriority=Speed  RndMeth=Simplest  InputSameDT=on
  driver look ahead seconds : Constant  Value=0.5
  limitedMCT : Lookup_n-D  NumberOfTableDimensions=1  BreakpointsForDimension1=limitedMCT.Time  Table=limitedMCT.Speed  InternalRulePriority=Speed  RndMeth=Simplest  InputSameDT=on
  pMCT : Lookup_n-D  NumberOfTableDimensions=1  BreakpointsForDimension1=pMCT.Time  Table=pMCT.Speed  InternalRulePriority=Speed  RndMeth=Simplest  InputSameDT=on
  DriverBus : Outport
  wires:
  Veh speed cycle trigger/1 -> Get Cycle Clock Time/1(Cycle Trigger)
  MCT/1 -> Multiport Switch/5
  US06/1 -> Multiport Switch/4
  Add/1 -> CoastDown/1, pMCT/1, limitedMCT/1, MCT/1, US06/1
  CoastDown/1 -> Multiport Switch/2
  pMCT/1 -> Multiport Switch/3
  DriveCycleSelect/1 -> Multiport Switch/1
  [VehSpdKph] -> Data Type Conversion11/1
  Driver and PI with FF Control/1(DriverBus) -> DriverBus/1
  Data Type Conversion11/1 -> Gain/1, Driver and PI with FF Control/1(Vehicle_Spd_kph)  "Vehicle_Spd_kph"
  Get Cycle Clock Time/1(tCycle) -> Add/2
  driver look ahead seconds/1 -> Add/1
  limitedMCT/1 -> Multiport Switch/6
  Veh speed feedback [kph]/1 -> [VehSpdKph]
  Gain/1 -> Scope/1, Terminator/1  "Vehicle_Spd_mph"
  Gain1/1 -> Scope/2, Terminator1/1  "Vehicle_SpdDmd_mph"
  Multiport Switch1/1 -> Gain1/1, Driver and PI with FF Control/2(Vehicle_SpdDmd_kph)  "RefSpd [km/hr]"
  Rate Limiter/1 -> Multiport Switch1/2
  ManSpdSel/1 -> Multiport Switch1/1
  Multiport Switch/1 -> Multiport Switch1/4
  Constant/1 -> Multiport Switch1/5
  [VehSpdKph] -> Multiport Switch1/3
  Pulse Generator/1 -> Rate Limiter/1

== system CAVE_MachE_sil_test_v2/Vehicle Under Test/Vehicle/From CAN ==
  BrakeSwitch : Inport
  Brake switch ource selection : Constant  Value=2
  Bus Creator1 : BusCreator  Inputs=2
  Demux : Demux  Outputs=1
  Ground : Ground
  Ground1 : Ground
  Multiport Switch1 : MultiPortSwitch  Inputs=2
  IO_Out : Outport
  wires:
  Bus Creator1/1 -> IO_Out/1  "IO_Out"
  Multiport Switch1/1 -> Bus Creator1/2  "BRAKE_LAMP_BOOL_CAN"
  Demux/1 -> Bus Creator1/1  "STEERING_ANGLE_DEG_CAN"
  Ground/1 -> Demux/1
  Brake switch ource selection/1 -> Multiport Switch1/1
  Ground1/1 -> Multiport Switch1/2  "Brake switch from CAN"
  BrakeSwitch/1 -> Multiport Switch1/3

== system CAVE_MachE_sil_test_v2/Vehicle Under Test/Vehicle/Front Wheel Drive ==
  DrvShfTrq : Inport
  Omega : Inport  Port=2
  Ideal Diff : Subsystem  VariantControl=0
  Ideal Diff AWD : Subsystem  VariantControl=Choice
  Real Diff : Subsystem  VariantControl=1
  Diff : Outport  VectorParamsAs1DForOutWhenUnconnected=off
  AxlTrq : Outport  Port=2  VectorParamsAs1DForOutWhenUnconnected=off
  PropShaftSpd : Outport  Port=3  VectorParamsAs1DForOutWhenUnconnected=off
